simulink model "MSM_strain_wave_actuator"  (R2024b)
settings: Solver=ode23t  StartTime=0.0  StopTime=SIMULATION_TIME  FixedStep=MAX_TIME_STEP  MaxStep=MAX_TIME_STEP  RelTol=1e-3  AbsTol=1e-3  EnableMultiTasking=on
PreLoadFcn:
  | linear_mechanism = Simulink.Variant('motion_type == "linear"');
  | rotary_mechanism = Simulink.Variant('motion_type == "rotary"');
values from neighbouring files (symbols this model uses):
  action = round(out.position_data.Data(:,5))    [msm_tooth_training_run.m]
  contact_ratio = tooth_plates_cnt / (2 * (t_a / t_b + 1))    (= 2)    [MSM_mechanism_simulation_properties.m]
  contraction_initial = -msm_length * e_initial    (= -0.001)    [MSM_mechanism_simulation_properties.m]
  controller_type_vec = zeros(tooth_plates_cnt, 1)    [MSM_mechanism_simulation_properties.m]
  controller_velocity_setpoint = velocity_iter    [controller_mass_comparison_runs.m]
  disk_diameter = disk_teeth_count * tooth_pitch / pi    [MSM_mechanism_simulation_properties.m]    (also in msm_sim_runs_for_pid.m = evalin('base','disk_diameter'); save_sim_result.m = evalin('base','disk_diameter'))
  disk_height = 2.5e-4    (= 0.00025)    [MSM_mechanism_simulation_properties.m]    (also in get_tooth_properties.m)
  feedback_threshold = 1.025    [MSM_mechanism_simulation_properties.m]    (also in get_tooth_properties.m; msm_sim_runs_for_pid.m = evalin('base','feedback_threshold'))
  force_control_coeff = 1.0    (= 1)    [MSM_mechanism_simulation_properties.m]
  HALT_VELOCITY = 0.2    [MSM_mechanism_simulation_properties.m]    (also in get_tooth_properties.m)
  in_pair_angle_tooth_plates_pitch = 2*pi * (-2*tooth_pitch + in_pair_tooth_plates_pitch) / (pi*disk_diameter)    (= 0.412285714286)    [MSM_mechanism_simulation_properties.m]    (also in get_tooth_properties.m = 2*pi * (-2*tooth_pitch + in_pair_tooth_plates_pitch) / (pi*t)
  MAX_OVERLOAD_VELOCITY = 100    [MSM_mechanism_simulation_properties.m]    (also in get_tooth_properties.m)
  MAX_POSITION = rack_initial_position + max_teeth_passed * tooth_plates_cnt * angle_single_tooth_step    [MSM_mechanism_simulation_properties.m]    (also in get_tooth_properties.m)
  MAX_TIME_STEP = 5e-6    (= 5e-06)    [MSM_mechanism_simulation_properties.m]
  min_tooth_motion_range = -msm_length * allowed_elongation    (= -0.001)    [MSM_mechanism_simulation_properties.m]
  motion_type_number = NaN    [MSM_mechanism_simulation_properties.m]
  next_vec_fraction = -0.05    [MSM_mechanism_simulation_properties.m]    (also in msm_sim_runs_for_pid.m = evalin('base','next_vec_fraction'))
  obs_matrix = zeros(tooth_plates_cnt, obs_matrix_size)    [MSM_mechanism_simulation_properties.m]
  one_side_absolute_offset = one_side_elongation_capacity * msm_length    (= 0.0001)    [MSM_mechanism_simulation_properties.m]
  rack_coulumb_friction = 0.05    [MSM_mechanism_simulation_properties.m]
  rack_initial_position = rack_initial_position + 4*angle_single_tooth_step    (= 0.0554357142857)    [MSM_mechanism_simulation_properties.m]    (also in get_tooth_properties.m = rack_initial_position + 4*angle_single_tooth_step)
  rack_mass = 4e-3    (= 0.004)    [MSM_mechanism_simulation_properties.m]
  rotational_rack_coulumb_friction = rack_coulumb_friction * disk_diameter    (= 0.00175)    [MSM_mechanism_simulation_properties.m]
  SIMULATION_TIME = 0.06    [MSM_mechanism_simulation_properties.m]    (also in msm_actuation_time_sensetivity.m = 0.04; msm_sim_runs_for_pid.m = evalin('base','SIMULATION_TIME'); msm_simulation_run.m = 0.08; msm_tooth_training_run.m = 0.04)
  swing_block_tooth_plates_pitch = 2 * tooth_pitch * 22 + tooth_pitch / tooth_plates_cnt    (= 0.0172575)    [MSM_mechanism_simulation_properties.m]    (also in get_tooth_properties.m = 2 * tooth_pitch * 22 + tooth_pitch / tooth_plates_cnt)
  tooth_disk_mass = 5e-3    (= 0.005)    [MSM_mechanism_simulation_properties.m]
  tooth_pitch = tooth_pitch * tooth_size_modifier    (= 0.00039)    [MSM_mechanism_simulation_properties.m]    (also in get_tooth_properties.m = 0.00024661; msm_sim_runs_for_pid.m = evalin('base','tooth_pitch'); save_sim_result.m = evalin('base','tooth_pitch'))
  tooth_plates_cnt = 4    [MSM_mechanism_simulation_properties.m]    (also in MSM_simulation_data_processing.m = sim_data.tooth_plates_cnt; msm_actuation_time_sensetivity.m = plates_cnt_iter; msm_sim_runs_for_pid.m = evalin('base','tooth_plates_cnt'); msm_simulation_run.m = plates_cnt_iter)
  tooth_plates_pitch = tooth_pitch * 12 + tooth_pitch / tooth_plates_cnt    (= 0.0047775)    [MSM_mechanism_simulation_properties.m]    (also in get_tooth_properties.m = tooth_pitch * 12 + tooth_pitch / tooth_plates_cnt)
  useful_load = -2    [MSM_mechanism_simulation_properties.m]    (also in controller_mass_comparison_runs.m)
  useful_mass = 0.0001    [MSM_mechanism_simulation_properties.m]    (also in controller_mass_comparison_runs.m = 0.025)
  VALIDATION_START_TIME = 0.25*SIMULATION_TIME    (= 0.015)    [MSM_mechanism_simulation_properties.m]
  Z = griddata(x,y,z,X,Y)    [MSM_simulation_data_processing.m]
undefined symbols (not defined in the file or in its folder): controller_amplitude_setpoint, controller_desired_profile_type, controller_frequency_setpoint, controller_loop_type, enable_neighbours_obs, enable_vel_setpoint, external_control_value, has_external_controller, initial_spike_force, random_delay_probablity, random_switch_probability, sim_state_code, simulation_pause_time, X, Y
libraries: sm_lib x141, MSM_element x72, Flat_tooth_plate x36, Rotary_tooth_plate x36, Swing_mechanism x18, nesl_utility x16, simulink x10, fl_lib x9, rllib x7, spsMeanLib x2, slctrl_autotuning x2, slpidlib x1
(part 6 of 7)

== system MSM_strain_wave_actuator/MSM elements variant subsystem/Variable plate count Rotary push push plates/Rotary push push 8 plates/Subsystem1 ==
  Control input [0; 1] : Inport
  Control input [0; 1]1 : Inport  Port=2
  Half pair rotation : sm_lib/Frames and Transforms/Rigid Transform  TranslationMethod=None  TranslationStandardOffset=0  TranslationStandardOffsetUnits=m  TranslationStandardAxis=+Z  TranslationCartesianOffset=[0 0 0]  TranslationCartesianOffsetUnits=m  TranslationROffset=0  TranslationROffsetUnits=m  TranslationZOffset=0  TranslationZOffsetUnits=m  TranslationThetaOffset=0  TranslationThetaOffsetUnits=deg  RotationMethod=StandardAxis  RotationAngleUnits=rad  RotationStandardAxis=+Z  RotationAngle=in_pair_angle_tooth_plates_pitch/2  RotationArbitraryAxis=[0 0 1]  FollAlignAxisA=+X  BaseAlignAxisA=+Y  FollAlignAxisB=+Y  BaseAlignAxisB=+Z  RotationSequenceAxes=FollowerAxes  RotationSequence=XYX  RotationSequenceAngles=[0 0 0]  RotationSequenceAnglesUnits=deg  RotationMatrix=[1 0 0; 0 1 0; 0 0 1]  Quaternion=[1 0 0 0]
  MSM and tooth plate1 : MSM_element/MSM and tooth plate  PositionTargetValue=contraction_initial * 0.4
  MSM and tooth plate2 : MSM_element/MSM and tooth plate  PositionTargetValue=contraction_initial * 0.6
  MSM plate translation1 : sm_lib/Frames and Transforms/Rigid Transform  TranslationMethod=StandardAxis  TranslationStandardOffset=disk_diameter / 2  TranslationStandardOffsetUnits=m  TranslationStandardAxis=+Y  TranslationCartesianOffset=[0 0 0]  TranslationCartesianOffsetUnits=m  TranslationROffset=0  TranslationROffsetUnits=m  TranslationZOffset=0  TranslationZOffsetUnits=m  TranslationThetaOffset=0  TranslationThetaOffsetUnits=deg  RotationMethod=StandardAxis  RotationAngleUnits=deg  RotationStandardAxis=-X  RotationAngle=90  RotationArbitraryAxis=[0 0 1]  FollAlignAxisA=+X  BaseAlignAxisA=+Y  FollAlignAxisB=+Y  BaseAlignAxisB=+Z  RotationSequenceAxes=FollowerAxes  RotationSequence=XYX  RotationSequenceAngles=[0 0 0]  RotationSequenceAnglesUnits=deg  RotationMatrix=[1 0 0; 0 1 0; 0 0 1]  Quaternion=[1 0 0 0]
  MSM plate translation2 : sm_lib/Frames and Transforms/Rigid Transform  TranslationMethod=StandardAxis  TranslationStandardOffset=disk_diameter / 2  TranslationStandardOffsetUnits=m  TranslationStandardAxis=+Y  TranslationCartesianOffset=[0 0 0]  TranslationCartesianOffsetUnits=m  TranslationROffset=0  TranslationROffsetUnits=m  TranslationZOffset=0  TranslationZOffsetUnits=m  TranslationThetaOffset=0  TranslationThetaOffsetUnits=deg  RotationMethod=StandardAxis  RotationAngleUnits=deg  RotationStandardAxis=-X  RotationAngle=90  RotationArbitraryAxis=[0 0 1]  FollAlignAxisA=+X  BaseAlignAxisA=+Y  FollAlignAxisB=+Y  BaseAlignAxisB=+Z  RotationSequenceAxes=FollowerAxes  RotationSequence=XYX  RotationSequenceAngles=[0 0 0]  RotationSequenceAnglesUnits=deg  RotationMatrix=[1 0 0; 0 1 0; 0 0 1]  Quaternion=[1 0 0 0]
  MSM plate translation4 : sm_lib/Frames and Transforms/Rigid Transform  TranslationMethod=StandardAxis  TranslationStandardOffset=disk_diameter / 2  TranslationStandardOffsetUnits=m  TranslationStandardAxis=+Y  TranslationCartesianOffset=[0 0 0]  TranslationCartesianOffsetUnits=m  TranslationROffset=0  TranslationROffsetUnits=m  TranslationZOffset=0  TranslationZOffsetUnits=m  TranslationThetaOffset=0  TranslationThetaOffsetUnits=deg  RotationMethod=StandardAxis  RotationAngleUnits=deg  RotationStandardAxis=-X  RotationAngle=90  RotationArbitraryAxis=[0 0 1]  FollAlignAxisA=+X  BaseAlignAxisA=+Y  FollAlignAxisB=+Y  BaseAlignAxisB=+Z  RotationSequenceAxes=FollowerAxes  RotationSequence=XYX  RotationSequenceAngles=[0 0 0]  RotationSequenceAnglesUnits=deg  RotationMatrix=[1 0 0; 0 1 0; 0 0 1]  Quaternion=[1 0 0 0]
  Rigid Transform1 : sm_lib/Frames and Transforms/Rigid Transform  TranslationMethod=None  TranslationStandardOffset=0  TranslationStandardOffsetUnits=m  TranslationStandardAxis=+Z  TranslationCartesianOffset=[0 0 0]  TranslationCartesianOffsetUnits=m  TranslationROffset=0  TranslationROffsetUnits=m  TranslationZOffset=0  TranslationZOffsetUnits=m  TranslationThetaOffset=0  TranslationThetaOffsetUnits=deg  RotationMethod=StandardAxis  RotationAngleUnits=rad  RotationStandardAxis=+Z  RotationAngle=in_pair_angle_tooth_plates_pitch  RotationArbitraryAxis=[0 0 1]  FollAlignAxisA=+X  BaseAlignAxisA=+Y  FollAlignAxisB=+Y  BaseAlignAxisB=+Z  RotationSequenceAxes=FollowerAxes  RotationSequence=XYX  RotationSequenceAngles=[0 0 0]  RotationSequenceAnglesUnits=deg  RotationMatrix=[1 0 0; 0 1 0; 0 0 1]  Quaternion=[1 0 0 0]
  Rotary_tooth_plate1 : Rotary_tooth_plate/Rotary_tooth_plate  SystemSampleTime=-1  VariantActivationTime=update diagram  AllowFlexibleInterface=on  Latency=0  AutoFrameSizeCalculation=off
  Rotary_tooth_plate2 : Rotary_tooth_plate/Rotary_tooth_plate  SystemSampleTime=-1  VariantActivationTime=update diagram  AllowFlexibleInterface=on  Latency=0  AutoFrameSizeCalculation=off
  Signal termination : sm_lib/Body Elements/Spherical Solid  GraphicAmbientColor=[0.15 0.15 0.15 1.0]  BasedOnType=Mass  CenterOfMass=[0 0 0]  CenterOfMassUnits=m  GraphicDiffuseColor=[0.5 0.5 0.5]  Density=1000  DensityUnits=kg/m^3  DoExposeReferenceFrame=on  GraphicEmissiveColor=[0.0 0.0 0.0 1.0]  ExportEntireGeometry=off  SerializedExposedGeometries=<ExposedGeometries/>  SerializedFrames=<Frames/>  MarkerShape=Sphere  MarkerSize=10  GraphicType=None  InertiaType=CalculateFromGeometry  Mass=1e-12  MassUnits=kg  MomentsOfInertia=[1 1 1]  MomentsOfInertiaUnits=kg*m^2  GraphicOpacity=1.0  ProductsOfInertia=[0 0 0]  ProductsOfInertiaUnits=kg*m^2  GraphicShininess=75  GraphicSpecularColor=[0.5 0.5 0.5 1.0]  SphereRadius=1  SphereRadiusUnits=m  GraphicVisPropType=SimpleVisualProperties
  Swing mechanism : Swing_mechanism/Swing mechanism  SystemSampleTime=-1  VariantActivationTime=update diagram  AllowFlexibleInterface=on  Latency=0  AutoFrameSizeCalculation=off
  Conn1 : PMIOPort  Side=Left
  Contact force : PMIOPort  Port=2  Side=Right
  "Tooth position, mm" : Outport
  "Tooth position, mm1" : Outport  Port=2
  wires:
  MSM and tooth plate2/1 -> "Tooth position, mm1"/1
  MSM and tooth plate1/1 -> "Tooth position, mm"/1
  Control input [0; 1]1/1 -> MSM and tooth plate2/1
  Control input [0; 1]/1 -> MSM and tooth plate1/1
  connections:
  Rotary_tooth_plate1/LConn2 -- MSM plate translation1/RConn1 -- MSM and tooth plate1/LConn1
  MSM and tooth plate2/RConn1 -- Swing mechanism/RConn1 -- Rotary_tooth_plate2/LConn1
  Rotary_tooth_plate1/RConn1 -- Rotary_tooth_plate2/RConn1 -- Contact force/RConn1
  Rigid Transform1/LConn1 -- Half pair rotation/LConn1 -- MSM plate translation1/LConn1 -- Conn1/RConn1
  MSM and tooth plate1/RConn1 -- Swing mechanism/RConn2 -- Rotary_tooth_plate1/LConn1
  MSM plate translation2/RConn1 -- Rotary_tooth_plate2/LConn2 -- MSM and tooth plate2/LConn1
  MSM plate translation4/RConn1 -- Swing mechanism/LConn1
  Half pair rotation/RConn1 -- MSM plate translation4/LConn1
  Rigid Transform1/RConn1 -- MSM plate translation2/LConn1
  Signal termination/RConn1 -- Swing mechanism/LConn2

== system MSM_strain_wave_actuator/MSM elements variant subsystem/Variable plate count Rotary push push plates/Rotary push push 8 plates/Subsystem2 ==
  Control input [0; 1] : Inport
  Control input [0; 1]1 : Inport  Port=2
  Half pair rotation : sm_lib/Frames and Transforms/Rigid Transform  TranslationMethod=None  TranslationStandardOffset=0  TranslationStandardOffsetUnits=m  TranslationStandardAxis=+Z  TranslationCartesianOffset=[0 0 0]  TranslationCartesianOffsetUnits=m  TranslationROffset=0  TranslationROffsetUnits=m  TranslationZOffset=0  TranslationZOffsetUnits=m  TranslationThetaOffset=0  TranslationThetaOffsetUnits=deg  RotationMethod=StandardAxis  RotationAngleUnits=rad  RotationStandardAxis=+Z  RotationAngle=in_pair_angle_tooth_plates_pitch/2  RotationArbitraryAxis=[0 0 1]  FollAlignAxisA=+X  BaseAlignAxisA=+Y  FollAlignAxisB=+Y  BaseAlignAxisB=+Z  RotationSequenceAxes=FollowerAxes  RotationSequence=XYX  RotationSequenceAngles=[0 0 0]  RotationSequenceAnglesUnits=deg  RotationMatrix=[1 0 0; 0 1 0; 0 0 1]  Quaternion=[1 0 0 0]
  MSM and tooth plate1 : MSM_element/MSM and tooth plate  PositionTargetValue=contraction_initial * 0.5
  MSM and tooth plate2 : MSM_element/MSM and tooth plate  PositionTargetValue=contraction_initial * 0.5
  MSM plate translation1 : sm_lib/Frames and Transforms/Rigid Transform  TranslationMethod=StandardAxis  TranslationStandardOffset=disk_diameter / 2  TranslationStandardOffsetUnits=m  TranslationStandardAxis=+Y  TranslationCartesianOffset=[0 0 0]  TranslationCartesianOffsetUnits=m  TranslationROffset=0  TranslationROffsetUnits=m  TranslationZOffset=0  TranslationZOffsetUnits=m  TranslationThetaOffset=0  TranslationThetaOffsetUnits=deg  RotationMethod=StandardAxis  RotationAngleUnits=deg  RotationStandardAxis=-X  RotationAngle=90  RotationArbitraryAxis=[0 0 1]  FollAlignAxisA=+X  BaseAlignAxisA=+Y  FollAlignAxisB=+Y  BaseAlignAxisB=+Z  RotationSequenceAxes=FollowerAxes  RotationSequence=XYX  RotationSequenceAngles=[0 0 0]  RotationSequenceAnglesUnits=deg  RotationMatrix=[1 0 0; 0 1 0; 0 0 1]  Quaternion=[1 0 0 0]
  MSM plate translation2 : sm_lib/Frames and Transforms/Rigid Transform  TranslationMethod=StandardAxis  TranslationStandardOffset=disk_diameter / 2  TranslationStandardOffsetUnits=m  TranslationStandardAxis=+Y  TranslationCartesianOffset=[0 0 0]  TranslationCartesianOffsetUnits=m  TranslationROffset=0  TranslationROffsetUnits=m  TranslationZOffset=0  TranslationZOffsetUnits=m  TranslationThetaOffset=0  TranslationThetaOffsetUnits=deg  RotationMethod=StandardAxis  RotationAngleUnits=deg  RotationStandardAxis=-X  RotationAngle=90  RotationArbitraryAxis=[0 0 1]  FollAlignAxisA=+X  BaseAlignAxisA=+Y  FollAlignAxisB=+Y  BaseAlignAxisB=+Z  RotationSequenceAxes=FollowerAxes  RotationSequence=XYX  RotationSequenceAngles=[0 0 0]  RotationSequenceAnglesUnits=deg  RotationMatrix=[1 0 0; 0 1 0; 0 0 1]  Quaternion=[1 0 0 0]
  MSM plate translation4 : sm_lib/Frames and Transforms/Rigid Transform  TranslationMethod=StandardAxis  TranslationStandardOffset=disk_diameter / 2  TranslationStandardOffsetUnits=m  TranslationStandardAxis=+Y  TranslationCartesianOffset=[0 0 0]  TranslationCartesianOffsetUnits=m  TranslationROffset=0  TranslationROffsetUnits=m  TranslationZOffset=0  TranslationZOffsetUnits=m  TranslationThetaOffset=0  TranslationThetaOffsetUnits=deg  RotationMethod=StandardAxis  RotationAngleUnits=deg  RotationStandardAxis=-X  RotationAngle=90  RotationArbitraryAxis=[0 0 1]  FollAlignAxisA=+X  BaseAlignAxisA=+Y  FollAlignAxisB=+Y  BaseAlignAxisB=+Z  RotationSequenceAxes=FollowerAxes  RotationSequence=XYX  RotationSequenceAngles=[0 0 0]  RotationSequenceAnglesUnits=deg  RotationMatrix=[1 0 0; 0 1 0; 0 0 1]  Quaternion=[1 0 0 0]
  Rigid Transform1 : sm_lib/Frames and Transforms/Rigid Transform  TranslationMethod=None  TranslationStandardOffset=0  TranslationStandardOffsetUnits=m  TranslationStandardAxis=+Z  TranslationCartesianOffset=[0 0 0]  TranslationCartesianOffsetUnits=m  TranslationROffset=0  TranslationROffsetUnits=m  TranslationZOffset=0  TranslationZOffsetUnits=m  TranslationThetaOffset=0  TranslationThetaOffsetUnits=deg  RotationMethod=StandardAxis  RotationAngleUnits=rad  RotationStandardAxis=+Z  RotationAngle=in_pair_angle_tooth_plates_pitch  RotationArbitraryAxis=[0 0 1]  FollAlignAxisA=+X  BaseAlignAxisA=+Y  FollAlignAxisB=+Y  BaseAlignAxisB=+Z  RotationSequenceAxes=FollowerAxes  RotationSequence=XYX  RotationSequenceAngles=[0 0 0]  RotationSequenceAnglesUnits=deg  RotationMatrix=[1 0 0; 0 1 0; 0 0 1]  Quaternion=[1 0 0 0]
  Rotary_tooth_plate1 : Rotary_tooth_plate/Rotary_tooth_plate  SystemSampleTime=-1  VariantActivationTime=update diagram  AllowFlexibleInterface=on  Latency=0  AutoFrameSizeCalculation=off
  Rotary_tooth_plate2 : Rotary_tooth_plate/Rotary_tooth_plate  SystemSampleTime=-1  VariantActivationTime=update diagram  AllowFlexibleInterface=on  Latency=0  AutoFrameSizeCalculation=off
  Signal termination : sm_lib/Body Elements/Spherical Solid  GraphicAmbientColor=[0.15 0.15 0.15 1.0]  BasedOnType=Mass  CenterOfMass=[0 0 0]  CenterOfMassUnits=m  GraphicDiffuseColor=[0.5 0.5 0.5]  Density=1000  DensityUnits=kg/m^3  DoExposeReferenceFrame=on  GraphicEmissiveColor=[0.0 0.0 0.0 1.0]  ExportEntireGeometry=off  SerializedExposedGeometries=<ExposedGeometries/>  SerializedFrames=<Frames/>  MarkerShape=Sphere  MarkerSize=10  GraphicType=None  InertiaType=CalculateFromGeometry  Mass=1e-12  MassUnits=kg  MomentsOfInertia=[1 1 1]  MomentsOfInertiaUnits=kg*m^2  GraphicOpacity=1.0  ProductsOfInertia=[0 0 0]  ProductsOfInertiaUnits=kg*m^2  GraphicShininess=75  GraphicSpecularColor=[0.5 0.5 0.5 1.0]  SphereRadius=1  SphereRadiusUnits=m  GraphicVisPropType=SimpleVisualProperties
  Swing mechanism : Swing_mechanism/Swing mechanism  SystemSampleTime=-1  VariantActivationTime=update diagram  AllowFlexibleInterface=on  Latency=0  AutoFrameSizeCalculation=off
  Conn1 : PMIOPort  Side=Left
  Contact force : PMIOPort  Port=2  Side=Right
  "Tooth position, mm" : Outport
  "Tooth position, mm1" : Outport  Port=2
  wires:
  MSM and tooth plate2/1 -> "Tooth position, mm1"/1
  MSM and tooth plate1/1 -> "Tooth position, mm"/1
  Control input [0; 1]1/1 -> MSM and tooth plate2/1
  Control input [0; 1]/1 -> MSM and tooth plate1/1
  connections:
  Rotary_tooth_plate1/LConn2 -- MSM plate translation1/RConn1 -- MSM and tooth plate1/LConn1
  MSM and tooth plate2/RConn1 -- Swing mechanism/RConn1 -- Rotary_tooth_plate2/LConn1
  Rotary_tooth_plate1/RConn1 -- Rotary_tooth_plate2/RConn1 -- Contact force/RConn1
  Rigid Transform1/LConn1 -- Half pair rotation/LConn1 -- MSM plate translation1/LConn1 -- Conn1/RConn1
  MSM and tooth plate1/RConn1 -- Swing mechanism/RConn2 -- Rotary_tooth_plate1/LConn1
  MSM plate translation2/RConn1 -- Rotary_tooth_plate2/LConn2 -- MSM and tooth plate2/LConn1
  MSM plate translation4/RConn1 -- Swing mechanism/LConn1
  Half pair rotation/RConn1 -- MSM plate translation4/LConn1
  Rigid Transform1/RConn1 -- MSM plate translation2/LConn1
  Signal termination/RConn1 -- Swing mechanism/LConn2

== system MSM_strain_wave_actuator/MSM elements variant subsystem/Variable plate count Rotary push push plates/Rotary push push 8 plates/Subsystem3 ==
  Control input [0; 1] : Inport
  Control input [0; 1]1 : Inport  Port=2
  Half pair rotation : sm_lib/Frames and Transforms/Rigid Transform  TranslationMethod=None  TranslationStandardOffset=0  TranslationStandardOffsetUnits=m  TranslationStandardAxis=+Z  TranslationCartesianOffset=[0 0 0]  TranslationCartesianOffsetUnits=m  TranslationROffset=0  TranslationROffsetUnits=m  TranslationZOffset=0  TranslationZOffsetUnits=m  TranslationThetaOffset=0  TranslationThetaOffsetUnits=deg  RotationMethod=StandardAxis  RotationAngleUnits=rad  RotationStandardAxis=+Z  RotationAngle=in_pair_angle_tooth_plates_pitch/2  RotationArbitraryAxis=[0 0 1]  FollAlignAxisA=+X  BaseAlignAxisA=+Y  FollAlignAxisB=+Y  BaseAlignAxisB=+Z  RotationSequenceAxes=FollowerAxes  RotationSequence=XYX  RotationSequenceAngles=[0 0 0]  RotationSequenceAnglesUnits=deg  RotationMatrix=[1 0 0; 0 1 0; 0 0 1]  Quaternion=[1 0 0 0]
  MSM and tooth plate1 : MSM_element/MSM and tooth plate  PositionTargetValue=contraction_initial * 0.7
  MSM and tooth plate2 : MSM_element/MSM and tooth plate  PositionTargetValue=contraction_initial * 0.3
  MSM plate translation1 : sm_lib/Frames and Transforms/Rigid Transform  TranslationMethod=StandardAxis  TranslationStandardOffset=disk_diameter / 2  TranslationStandardOffsetUnits=m  TranslationStandardAxis=+Y  TranslationCartesianOffset=[0 0 0]  TranslationCartesianOffsetUnits=m  TranslationROffset=0  TranslationROffsetUnits=m  TranslationZOffset=0  TranslationZOffsetUnits=m  TranslationThetaOffset=0  TranslationThetaOffsetUnits=deg  RotationMethod=StandardAxis  RotationAngleUnits=deg  RotationStandardAxis=-X  RotationAngle=90  RotationArbitraryAxis=[0 0 1]  FollAlignAxisA=+X  BaseAlignAxisA=+Y  FollAlignAxisB=+Y  BaseAlignAxisB=+Z  RotationSequenceAxes=FollowerAxes  RotationSequence=XYX  RotationSequenceAngles=[0 0 0]  RotationSequenceAnglesUnits=deg  RotationMatrix=[1 0 0; 0 1 0; 0 0 1]  Quaternion=[1 0 0 0]
  MSM plate translation2 : sm_lib/Frames and Transforms/Rigid Transform  TranslationMethod=StandardAxis  TranslationStandardOffset=disk_diameter / 2  TranslationStandardOffsetUnits=m  TranslationStandardAxis=+Y  TranslationCartesianOffset=[0 0 0]  TranslationCartesianOffsetUnits=m  TranslationROffset=0  TranslationROffsetUnits=m  TranslationZOffset=0  TranslationZOffsetUnits=m  TranslationThetaOffset=0  TranslationThetaOffsetUnits=deg  RotationMethod=StandardAxis  RotationAngleUnits=deg  RotationStandardAxis=-X  RotationAngle=90  RotationArbitraryAxis=[0 0 1]  FollAlignAxisA=+X  BaseAlignAxisA=+Y  FollAlignAxisB=+Y  BaseAlignAxisB=+Z  RotationSequenceAxes=FollowerAxes  RotationSequence=XYX  RotationSequenceAngles=[0 0 0]  RotationSequenceAnglesUnits=deg  RotationMatrix=[1 0 0; 0 1 0; 0 0 1]  Quaternion=[1 0 0 0]
  MSM plate translation4 : sm_lib/Frames and Transforms/Rigid Transform  TranslationMethod=StandardAxis  TranslationStandardOffset=disk_diameter / 2  TranslationStandardOffsetUnits=m  TranslationStandardAxis=+Y  TranslationCartesianOffset=[0 0 0]  TranslationCartesianOffsetUnits=m  TranslationROffset=0  TranslationROffsetUnits=m  TranslationZOffset=0  TranslationZOffsetUnits=m  TranslationThetaOffset=0  TranslationThetaOffsetUnits=deg  RotationMethod=StandardAxis  RotationAngleUnits=deg  RotationStandardAxis=-X  RotationAngle=90  RotationArbitraryAxis=[0 0 1]  FollAlignAxisA=+X  BaseAlignAxisA=+Y  FollAlignAxisB=+Y  BaseAlignAxisB=+Z  RotationSequenceAxes=FollowerAxes  RotationSequence=XYX  RotationSequenceAngles=[0 0 0]  RotationSequenceAnglesUnits=deg  RotationMatrix=[1 0 0; 0 1 0; 0 0 1]  Quaternion=[1 0 0 0]
  Rigid Transform1 : sm_lib/Frames and Transforms/Rigid Transform  TranslationMethod=None  TranslationStandardOffset=0  TranslationStandardOffsetUnits=m  TranslationStandardAxis=+Z  TranslationCartesianOffset=[0 0 0]  TranslationCartesianOffsetUnits=m  TranslationROffset=0  TranslationROffsetUnits=m  TranslationZOffset=0  TranslationZOffsetUnits=m  TranslationThetaOffset=0  TranslationThetaOffsetUnits=deg  RotationMethod=StandardAxis  RotationAngleUnits=rad  RotationStandardAxis=+Z  RotationAngle=in_pair_angle_tooth_plates_pitch  RotationArbitraryAxis=[0 0 1]  FollAlignAxisA=+X  BaseAlignAxisA=+Y  FollAlignAxisB=+Y  BaseAlignAxisB=+Z  RotationSequenceAxes=FollowerAxes  RotationSequence=XYX  RotationSequenceAngles=[0 0 0]  RotationSequenceAnglesUnits=deg  RotationMatrix=[1 0 0; 0 1 0; 0 0 1]  Quaternion=[1 0 0 0]
  Rotary_tooth_plate1 : Rotary_tooth_plate/Rotary_tooth_plate  SystemSampleTime=-1  VariantActivationTime=update diagram  AllowFlexibleInterface=on  Latency=0  AutoFrameSizeCalculation=off
  Rotary_tooth_plate2 : Rotary_tooth_plate/Rotary_tooth_plate  SystemSampleTime=-1  VariantActivationTime=update diagram  AllowFlexibleInterface=on  Latency=0  AutoFrameSizeCalculation=off
  Signal termination : sm_lib/Body Elements/Spherical Solid  GraphicAmbientColor=[0.15 0.15 0.15 1.0]  BasedOnType=Mass  CenterOfMass=[0 0 0]  CenterOfMassUnits=m  GraphicDiffuseColor=[0.5 0.5 0.5]  Density=1000  DensityUnits=kg/m^3  DoExposeReferenceFrame=on  GraphicEmissiveColor=[0.0 0.0 0.0 1.0]  ExportEntireGeometry=off  SerializedExposedGeometries=<ExposedGeometries/>  SerializedFrames=<Frames/>  MarkerShape=Sphere  MarkerSize=10  GraphicType=None  InertiaType=CalculateFromGeometry  Mass=1e-12  MassUnits=kg  MomentsOfInertia=[1 1 1]  MomentsOfInertiaUnits=kg*m^2  GraphicOpacity=1.0  ProductsOfInertia=[0 0 0]  ProductsOfInertiaUnits=kg*m^2  GraphicShininess=75  GraphicSpecularColor=[0.5 0.5 0.5 1.0]  SphereRadius=1  SphereRadiusUnits=m  GraphicVisPropType=SimpleVisualProperties
  Swing mechanism : Swing_mechanism/Swing mechanism  SystemSampleTime=-1  VariantActivationTime=update diagram  AllowFlexibleInterface=on  Latency=0  AutoFrameSizeCalculation=off
  Conn1 : PMIOPort  Side=Left
  Contact force : PMIOPort  Port=2  Side=Right
  "Tooth position, mm" : Outport
  "Tooth position, mm1" : Outport  Port=2
  wires:
  MSM and tooth plate2/1 -> "Tooth position, mm1"/1
  MSM and tooth plate1/1 -> "Tooth position, mm"/1
  Control input [0; 1]1/1 -> MSM and tooth plate2/1
  Control input [0; 1]/1 -> MSM and tooth plate1/1
  connections:
  Rotary_tooth_plate1/LConn2 -- MSM plate translation1/RConn1 -- MSM and tooth plate1/LConn1
  MSM and tooth plate2/RConn1 -- Swing mechanism/RConn1 -- Rotary_tooth_plate2/LConn1
  Rotary_tooth_plate1/RConn1 -- Rotary_tooth_plate2/RConn1 -- Contact force/RConn1
  Rigid Transform1/LConn1 -- Half pair rotation/LConn1 -- MSM plate translation1/LConn1 -- Conn1/RConn1
  MSM and tooth plate1/RConn1 -- Swing mechanism/RConn2 -- Rotary_tooth_plate1/LConn1
  MSM plate translation2/RConn1 -- Rotary_tooth_plate2/LConn2 -- MSM and tooth plate2/LConn1
  MSM plate translation4/RConn1 -- Swing mechanism/LConn1
  Half pair rotation/RConn1 -- MSM plate translation4/LConn1
  Rigid Transform1/RConn1 -- MSM plate translation2/LConn1
  Signal termination/RConn1 -- Swing mechanism/LConn2

== system MSM_strain_wave_actuator/controller/Old controller/Check if actuator halted or overloaded or reached max position1/Save scalar result ==
  stop_sim_code : Inport
  Enable : EnablePort
  To Workspace : ToWorkspace  VariableName=sim_stop_result  SaveFormat=Timeseries  SampleTime=-1
  wires:
  stop_sim_code/1 -> To Workspace/1

== matlab function MSM_strain_wave_actuator/Rack type variant subsystem/Rotary_gear/Single element frequency ==
  data: time input; cur_rack_position input; frequency output; rack_initial_position parameter; tooth_pitch parameter; disk_diameter parameter
function frequency = fcn(time, cur_rack_position, rack_initial_position, tooth_pitch, disk_diameter)
% frequncy in Hz


if time < 1e-3
    frequency = 0;
    return;
end


frequency = abs(cur_rack_position - rack_initial_position) / time / (2 * tooth_pitch / disk_diameter);

== matlab function MSM_strain_wave_actuator/controller/Control signals selector ==
  data: nn_input input; control_signal output; analytic_input input; selector_vec input; tooth_plates_cnt parameter
function control_signal = fcn(nn_input, analytic_input, selector_vec,...
    tooth_plates_cnt) % params
% The function selects control typåe for each individual tooth
% selector_vec - size = tooth_plates_cnt, if vec element is 1 or more, the
% nn_input is selected, otherwise the analytical input is selected

control_signal = analytic_input;
for i = 1 : tooth_plates_cnt
    if selector_vec(i) > 0.5
        control_signal(i) = nn_input(i);
    end
end

== matlab function MSM_strain_wave_actuator/controller/reward function ==
  data: stop_sim_code input; rack_abs_pos input; instant_rack_vel input; controller_velocity_setpoint input; reward output; isdone output; tooth_plates_cnt parameter; sim_state_code parameter; rack_initial_position parameter; enable_vel_setpoint parameter
function [reward,isdone] = reward(stop_sim_code, rack_abs_pos, instant_rack_vel,  controller_velocity_setpoint,...
    tooth_plates_cnt, sim_state_code, rack_initial_position, enable_vel_setpoint) % params

%instant_rack_vel = observation(3 * tooth_plates_cnt + 2);

% if time < 1e-7
%     rack_vel = instant_rack_vel;
% else
%     rack_vel = -rack_abs_pos / time; % measuring rack average velocity; Negative value taken
% end

% calculate reward value
reward = 0;

% penalty for staying still:
% if abs(instant_rack_vel) < 0.001
%     reward = reward - 1;
% end
% if instant_rack_vel > -0.001
%     reward = reward - 0.2;
% end

% if sum(action > 0.5) > 0.75 * tooth_plates_cnt
%     reward = reward - 10; % punish for too many active MSM elements at a time
% end
if enable_vel_setpoint % the reward is computed differently in case a velocity setpoint is followed
    reward = -sqrt(abs(instant_rack_vel - controller_velocity_setpoint)); % in ideal case reward is zero
end

if stop_sim_code ~= sim_state_code.SIM_OK
    if stop_sim_code == sim_state_code.SIM_MAX_POS_REACHED  % bonus for speed
        reward = reward + 20; % TODO correct value
    elseif stop_sim_code == sim_state_code.SIM_MAX_TIME_REACHED
        reward = reward + 0; % no bonus points for timeout so far. should there be some?
    else  % either in halt or overload states
        reward = reward - 20;
    end
end 

% done if either failed (crashed) or succeeded
isdone = boolean(stop_sim_code);

== matlab function MSM_strain_wave_actuator/controller/Timing PID controller/PID controller ==
  data: feedback input; control_vec output
function control_vec = fcn(feedback)
% feedback = (rack_pos, rack_vel, rack_acc, desired_vel)


control_vec = [1 0];

== matlab function MSM_strain_wave_actuator/ /initial spike force decay ==
  data: spike_force input; spike_force_output output; prev_value input
function spike_force_output = fcn(spike_force, prev_value)

if abs(prev_value) > 1e-6
    spike_force_output = 0;
else
    spike_force_output = spike_force;
end

== matlab function MSM_strain_wave_actuator/ /MATLAB Function ==
  data: feedback_input input; useful_load input; initial_spike_force input; load output; initial_spike output; is_load_applied output; prev_state input
function [load, initial_spike, is_load_applied] = fcn(feedback_input, useful_load, initial_spike_force, prev_state)

load = 0;
initial_spike = 0;
is_load_applied = 0;
if prev_state < 0.5 
    if max(feedback_input) > 0.5
        is_load_applied = 1;
        initial_spike = 1;
        load = initial_spike_force;
    end
else
    is_load_applied = 1;
    load = useful_load;
end

== matlab function MSM_strain_wave_actuator/controller/Controller output randomizer ==
  settings: updateMethod=DISCRETE
  data: control_input input; control_output output; previous_control_input input; random_delay_probablity parameter; random_switch_probability parameter; tooth_plates_cnt parameter
function control_output = fcn(control_input, previous_control_input, ...
    random_delay_probablity, random_switch_probability, tooth_plates_cnt) % params
% implements a random delay on controller action, additionally changes
% output randomly

control_output = control_input;

for i = 1 : tooth_plates_cnt
    if rand < random_switch_probability
        control_output(i) = xor(round(control_input(i)), 1); % flipping the controller output value
    elseif control_input(i) ~= previous_control_input(i) && rand < random_delay_probablity
        control_output(i) = previous_control_input(i);
    end
end

== matlab function MSM_strain_wave_actuator/controller/Old controller/Check if actuator halted or overloaded or reached max position1/Check sim stop conditions ==
  data: is_load_applied input; time input; stop_sim_code output; rack_velocity output; out_pos output; rack_cur_pos input; memory_pos input; MAX_OVERLOAD_VELOCITY parameter; HALT_VELOCITY parameter; SIMULATION_TIME parameter; MAX_POSITION parameter; VALIDATION_START_TIME parameter; rack_initial_position parameter; sim_state_code parameter
function [stop_sim_code, rack_velocity, out_pos] = fcn(is_load_applied, time, rack_cur_pos, memory_pos, ...
    MAX_OVERLOAD_VELOCITY, HALT_VELOCITY, SIMULATION_TIME,... % parameters are on this line
    MAX_POSITION, VALIDATION_START_TIME, rack_initial_position, sim_state_code) % parameters are on this line
% the function detects if the rack is not moving or overloaded and sends
% the corresponding code as the output
% see stop sim codes descriptions in the matlab properties file
%validation_start_time = 0.05*SIMULATION_TIME;
rack_velocity = 0;
if isnan(memory_pos) && time > 0.6*VALIDATION_START_TIME  % memorizing the initial rack state, 0.5 is good for linear
    out_pos = rack_cur_pos;
else
    out_pos = memory_pos;
end

stop_sim_code = sim_state_code.SIM_OK;  % 0 == not stopping the simulation
if ~is_load_applied || time < VALIDATION_START_TIME
    return
end

rack_velocity = abs(rack_cur_pos - memory_pos) / time;
if rack_velocity > MAX_OVERLOAD_VELOCITY % abs(rack_cur_pos - memory_pos) / time > MAX_OVERLOAD_VELOCITY
    stop_sim_code = sim_state_code.SIM_OVERLOAD;
    return;
end

if  rack_velocity < HALT_VELOCITY
    stop_sim_code = sim_state_code.SIM_HALT;
    return;
end

if abs(rack_cur_pos - rack_initial_position) > MAX_POSITION
    stop_sim_code = sim_state_code.SIM_MAX_POS_REACHED;
    return;
end

if time > SIMULATION_TIME
    stop_sim_code = sim_state_code.SIM_MAX_TIME_REACHED;
    return;
end

== matlab function MSM_strain_wave_actuator/controller/Old controller/Closed//open loop simple feedback controller1/MATLAB Function ==
  data: time input; output_vector output; loop_type input; cycle_length input; initial_idle_time input; feedback input; rack_position input; ticks_cnt input; currently_active input; tooth_plates_cnt parameter; cur_active_output output; feedback_threshold parameter; tooth_pitch parameter; rack_initial_position parameter; disk_diameter parameter; motion_type_number parameter; contact_ratio parameter; next_vec_fraction parameter
function [output_vector, cur_active_output]   = fcn(time, loop_type, cycle_length, ... % open loop inputs
    initial_idle_time, ... % input for stable simulation data
    feedback, rack_position,  ticks_cnt, currently_active,... % closed loop inputs (two different feedback methods)
    tooth_plates_cnt, feedback_threshold, tooth_pitch, rack_initial_position, disk_diameter, motion_type_number, contact_ratio, next_vec_fraction)  % this line contains parameters

% loop_type - lower than 0.5 is open loop, any value higher than 0.5 is a closed loop
% open loop parameters:
% cycle_length - duration of the actuation cycle of the whole plate set
% closed loop parameters:
% feedback, position feedback in range [0, 1], where 0 is fully contracted and 1 is fully extended
% motion_type_number: 0 == linear, 1 == rotary.
% next_vec_fraction - defines the disengagement timing for the last tooth,
% Positive value leads to earlier disengagement and negative value to the later disengagement

output_vector = zeros(tooth_plates_cnt, 1);
cur_active_output = currently_active;
tick = 0;

if time < initial_idle_time; return; end

if loop_type < 0.5 % open loop
    frac = mod(abs(time / cycle_length), 1);
    cur_active = -1;
    for i = 1:tooth_plates_cnt
        if frac < i / tooth_plates_cnt
            output_vector(i) = 1;
            if currently_active ~= i; tick = 1; end
            cur_active = i;
            cur_active_output = i;
            break;
        end
    end
    %if ticks_cnt > 0.5
    output_vector(cur_active_output) = 1; % this line added without testing. TODO test if it works properly
    output_vector(get_following_active_vec(cur_active, tooth_plates_cnt)) = 1; % TODO: modify open loop to support contact ratio
    %end
    return;
end

% ===== closed loop section =====

% next_active_vec = get_following_active_vec(currently_active, tooth_plates_cnt);

% --- Feedbacks based on complition of extension of a previous MSM element
% (so the next element is considered as "active"

% - original switch:
% if feedback(currently_active) > feedback_threshold %% 0.9 for the big pitch, over 0.9 for the small pitch
%     cur_active_output = next_active_vec(1);
%     tick = 1;
% end

% - modified switch: --- has problems at low loads where several active
% elements start to compete with each other
% for i = 1 : tooth_plates_cnt
%     if feedback(i) > feedback_threshold %% 0.9 for the big pitch, over 0.9 for the small pitch
%         tmp_next_active = get_following_active_vec(i, tooth_plates_cnt);
%         cur_active_output = tmp_next_active(1);
%         next_active_vec = get_following_active_vec(tmp_next_active(1), tooth_plates_cnt);
%         tick = 1;
%     end
% end


% --- rack feedback ---  Active element is determined based on the rack/disk position

% next_vec_fraction = 0; % before next_vec_fraction was a parameter, it had been defined on this line
for i = 2 : tooth_plates_cnt + 1
    if motion_type_number == 0 % linear case
        cur_cycle = rem(abs(rack_position - rack_initial_position - tooth_pitch), tooth_pitch); % getting reminder of the division. the substraction of the extra tooth_pitch is needed to guarantee first element push at the initial state
        switch_threshold = (i - 1) * tooth_pitch / tooth_plates_cnt - (1 - feedback_threshold) * tooth_pitch / tooth_plates_cnt; % the second term is to eliminate dead points
    else % rotary case % fi_max = 2*tooth_pitch / disk_diameter;  % - 2*tooth_pitch / disk_diameter
        cur_cycle = rem(abs(rack_position - rack_initial_position + 2*tooth_pitch / disk_diameter), 2*tooth_pitch / disk_diameter); % the extra addition of 2*tooth_pitch / disk_diamete has the same logic as for linear case (see the comments above)
        switch_threshold = (i - 1) * 2 * tooth_pitch / tooth_plates_cnt / disk_diameter - (1 - feedback_threshold) * 2 * tooth_pitch / tooth_plates_cnt / disk_diameter;
    end
    if cur_cycle < switch_threshold || i == tooth_plates_cnt + 1 % the second condition is a new part
        if i == tooth_plates_cnt + 1
            i = 1;
        end
        currently_active = i;
        cur_active_output = i; % questionable
        break
    end
end

next_active_vec = get_following_active_vec(currently_active, tooth_plates_cnt, contact_ratio, next_vec_fraction); % CR is concidered
% next_active_vec = get_following_active_vec(currently_active, tooth_plates_cnt); % this call always engages 50% of the teeth

% if ticks_cnt > 0.5
output_vector(next_active_vec) = 1;
% end
output_vector(cur_active_output) = 1;
% if ticks_cnt > 0.5
%     cur_active_output = next_active_vec(1);
% end

end

function following_active_vec = get_following_active_vec(cur_active, plates_cnt, contact_ratio, fraction)
% fraction - optional; is in [0; 1] range
% contact_ratio - optional; if contact ratio is unknown, the N/2 value can be used with 0 fraction.
% The performance will be higher if the contact ration is given. (N = tooth_plates_cnt)
    if nargin < 3
        iteration_range = cur_active + 1 : cur_active + round(plates_cnt / 2) - 1; % cur_active + ceil(plates_cnt / 2) - 1
    else
        fraction_tooth = ceil(mod(contact_ratio, 1) - fraction - 1e-6);
        % if fraction_tooth < 0; fraction_tooth = 0; end  % in case fraction ratio is too big. this line has been never tested
        iteration_range = cur_active + 1 : cur_active + round(floor(contact_ratio)) - 1 + fraction_tooth;
    end
    following_active_vec = 1:0; % creating empty double vector with this line, otherwise matlab will show a data cast warning later 
    for i = 1:length(iteration_range) % otherwise the Matlab coder does not work
        new_active_val = mod(iteration_range(i), plates_cnt+1);
        if new_active_val < cur_active
            new_active_val = new_active_val + 1;
        end
        following_active_vec = [following_active_vec new_active_val];
    end
end

== matlab function MSM_strain_wave_actuator/controller/Old controller/Control signals selector1 ==
  data: nn_input input; control_signal output; analytic_input input; selector_vec input; tooth_plates_cnt parameter
function control_signal = fcn(nn_input, analytic_input, selector_vec,...
    tooth_plates_cnt) % params
% The function selects control typåe for each individual tooth
% selector_vec - size = tooth_plates_cnt, if vec element is 1 or more, the
% nn_input is selected, otherwise the analytical input is selected

control_signal = analytic_input;
for i = 1 : tooth_plates_cnt
    if selector_vec(i) > 0.5
        control_signal(i) = nn_input(i);
    end
end

== matlab function MSM_strain_wave_actuator/controller/Old controller/Controller output randomizer1 ==
  settings: updateMethod=DISCRETE
  data: control_input input; control_output output; previous_control_input input; random_delay_probablity parameter; random_switch_probability parameter; tooth_plates_cnt parameter
function control_output = fcn(control_input, previous_control_input, ...
    random_delay_probablity, random_switch_probability, tooth_plates_cnt) % params
% implements a random delay on controller action, additionally changes
% output randomly

control_output = control_input;

for i = 1 : tooth_plates_cnt
    if rand < random_switch_probability
        control_output(i) = xor(round(control_input(i)), 1); % flipping the controller output value
    elseif control_input(i) ~= previous_control_input(i) && rand < random_delay_probablity
        control_output(i) = previous_control_input(i);
    end
end

== matlab function MSM_strain_wave_actuator/controller/Old controller/map observations to matrix1 ==
  data: tooth_pos input; vec_1 output; d1_tooth_pos input; d2_tooth_pos input; abs_rack_pos input; rack_vel input; rack_acc input; vel_setpoint input; tooth_plates_cnt parameter; tooth_pitch parameter; rack_initial_position parameter; vec_2 output; vec_3 output; vec_4 output; enable_neighbours_obs parameter; enable_vel_setpoint parameter; obs_matrix parameter
function [vec_1, vec_2, vec_3, vec_4]  = fcn(tooth_pos, d1_tooth_pos, d2_tooth_pos, abs_rack_pos, rack_vel, rack_acc, ...
    vel_setpoint,... % desired velocity setpoint
    tooth_plates_cnt, tooth_pitch, rack_initial_position,... % params here and next
    enable_neighbours_obs, ...  % flag, if > 0.5 the observation output also includes pos and vel data of neightbouring elements 
    enable_vel_setpoint,... % flag, if > 0.5 the observation output also includes velocity setpoint value, provided in vel_setpoin argument
    obs_matrix)

% obs_matrix - matrix in which observation for a particular tooth
% corresponds with a certain row
% separate vectors are output because it is not possible to select and feed
% correcsponding vector from the obs_matrix using "Variable Selector" block
obs_matrix(:, :) = 0; % erasing previously recorded values

for i = 1 : tooth_plates_cnt
    offset_rack_pos = abs_rack_pos - rack_initial_position - (i-1) * tooth_pitch / tooth_plates_cnt;
    if offset_rack_pos > 0
        teeth_offset_to_positive = ceil(offset_rack_pos / tooth_pitch); %floor
        offset_rack_pos = offset_rack_pos - abs(teeth_offset_to_positive) * tooth_pitch;
    end
    relavitve_rack_pos = rem(abs(offset_rack_pos), tooth_pitch) / tooth_pitch; % substraction of (i-1)... is to make; % rem(abs(abs_rack_pos - rack_initial_position - (i-1) * tooth_pitch / tooth_plates_cnt) , tooth_pitch) / tooth_pitch;
    % the system work correctly at the negative rack pos, however positive coordinates in this case are not validated
    obs_matrix(i, 1:6) = [tooth_pos(i) d1_tooth_pos(i) d2_tooth_pos(i) relavitve_rack_pos rack_vel rack_acc];
    if enable_neighbours_obs > 0.5  % include observations of neighbours pos and velocity
        [idx1, idx2] =  get_neighbour_index(i, tooth_plates_cnt);
        obs_matrix(i, 7) = tooth_pos(idx1);
        obs_matrix(i, 8) = d1_tooth_pos(idx1);
        obs_matrix(i, 9) = tooth_pos(idx2);
        obs_matrix(i, 10) = d1_tooth_pos(idx2);
    end
    if enable_vel_setpoint > 0.5
        obs_matrix(i, end) = vel_setpoint;
    end
end

vec_1 = obs_matrix(1, :)';
vec_2 = obs_matrix(2, :)';
vec_3 = obs_matrix(3, :)';
vec_4 = obs_matrix(4, :)';

end


function [idx1, idx2] =  get_neighbour_index(cur_idx, tooth_plates_cnt)
% returns the indexes of surrounding elements
idx1 = cur_idx - 1;
idx2 = cur_idx + 1;
if idx1 < 1
    idx1 = tooth_plates_cnt;
end
if idx2 > tooth_plates_cnt
    idx2 = 1;
end

end

== matlab function MSM_strain_wave_actuator/controller/Old controller/reward function1 ==
  data: observation input; stop_sim_code input; rack_abs_pos input; instant_rack_vel input; time input; action input; controller_velocity_setpoint input; reward output; isdone output; tooth_plates_cnt parameter; sim_state_code parameter; rack_initial_position parameter; enable_vel_setpoint parameter
function [reward,isdone] = reward(observation, stop_sim_code, rack_abs_pos, instant_rack_vel, time, action, controller_velocity_setpoint,...
    tooth_plates_cnt, sim_state_code, rack_initial_position, enable_vel_setpoint) % params

%instant_rack_vel = observation(3 * tooth_plates_cnt + 2);

% if time < 1e-7
%     rack_vel = instant_rack_vel;
% else
%     rack_vel = -rack_abs_pos / time; % measuring rack average velocity; Negative value taken
% end
% not in use as tanh is the output func
% action_regularization = sum(action > 1) + sum(action > 0);  % if the NN outputs too high control actions it results in penalty

% calculate reward value
% reward = rack_vel + 0.001*instant_rack_vel;
reward =  - instant_rack_vel - (rack_abs_pos - rack_initial_position);

% penalty for staying still:
% if abs(instant_rack_vel) < 0.001
%     reward = reward - 1;
% end
if instant_rack_vel > -0.001
    reward = reward - 0.2;
end

% if sum(action > 0.5) > 0.75 * tooth_plates_cnt
%     reward = reward - 10; % punish for too many active MSM elements at a time
% end
if enable_vel_setpoint % the reward is computed differently in case a velocity setpoint is followed
    reward = -sqrt(abs(instant_rack_vel - controller_velocity_setpoint)); % in ideal case reward is zero
end

if stop_sim_code ~= sim_state_code.SIM_OK
    if stop_sim_code == sim_state_code.SIM_MAX_POS_REACHED  % bonus for speed
        reward = reward + 20; % TODO correct value
    elseif stop_sim_code == sim_state_code.SIM_MAX_TIME_REACHED
        reward = reward + 0; % no bonus points for timeout so far. should there be some?
    else  % either in halt or overload states
        reward = reward - 20;
    end
end 

% done if either failed (crashed) or succeeded
isdone = boolean(stop_sim_code);

== matlab function MSM_strain_wave_actuator/controller/Check if actuator halted or overloaded or reached max position/Check sim stop conditions ==
  data: is_load_applied input; time input; stop_sim_code output; rack_velocity output; out_pos output; rack_cur_pos input; memory_pos input; MAX_OVERLOAD_VELOCITY parameter; HALT_VELOCITY parameter; SIMULATION_TIME parameter; MAX_POSITION parameter; VALIDATION_START_TIME parameter; rack_initial_position parameter; sim_state_code parameter
function [stop_sim_code, rack_velocity, out_pos] = fcn(is_load_applied, time, rack_cur_pos, memory_pos, ...
    MAX_OVERLOAD_VELOCITY, HALT_VELOCITY, SIMULATION_TIME,... % parameters are on this line
    MAX_POSITION, VALIDATION_START_TIME, rack_initial_position, sim_state_code) % parameters are on this line
% the function detects if the rack is not moving or overloaded and sends
% the corresponding code as the output
% see stop sim codes descriptions in the matlab properties file
%validation_start_time = 0.05*SIMULATION_TIME;
rack_velocity = 0;
if isnan(memory_pos) && time > 0.6*VALIDATION_START_TIME  % memorizing the initial rack state, 0.5 is good for linear
    out_pos = rack_cur_pos;
else
    out_pos = memory_pos;
end

stop_sim_code = sim_state_code.SIM_OK;  % 0 == not stopping the simulation
if ~is_load_applied || time < VALIDATION_START_TIME
    return
end

rack_velocity = abs(rack_cur_pos - memory_pos) / time;
if rack_velocity > MAX_OVERLOAD_VELOCITY % abs(rack_cur_pos - memory_pos) / time > MAX_OVERLOAD_VELOCITY
    stop_sim_code = sim_state_code.SIM_OVERLOAD;
    return;
end

if  rack_velocity < HALT_VELOCITY
    stop_sim_code = sim_state_code.SIM_HALT;
    return;
end

if abs(rack_cur_pos - rack_initial_position) > MAX_POSITION
    stop_sim_code = sim_state_code.SIM_MAX_POS_REACHED;
    return;
end

if time > SIMULATION_TIME
    stop_sim_code = sim_state_code.SIM_MAX_TIME_REACHED;
    return;
end
